simulink model "tasks"  (R2018a)
settings: Solver=FixedStepAuto  StartTime=0.0  StopTime=30  FixedStep=0.01  RelTol=1e-3
undefined symbols (not defined in the file): sigbuilder_block
settings Model: EnablePacing=on  Creator=U500304  LastModifiedBy=U500304

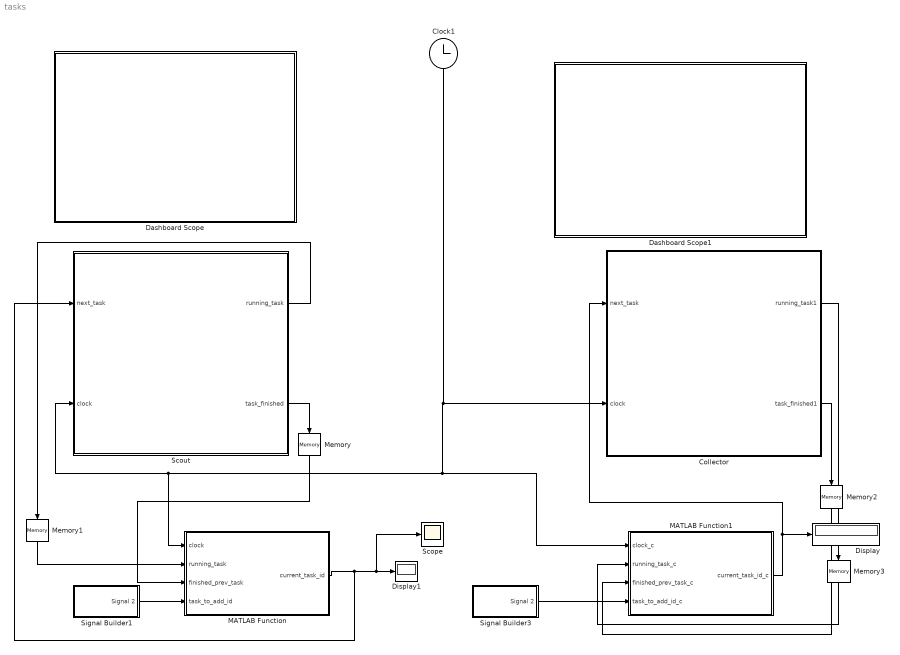
== system tasks ==
  Clock1 : Clock
  "Collector " : Subsystem
  Dashboard Scope : Subsystem  DialogController=hmiCreateDDGDialog  IsWebBlock=on  mask(MWDashboardBlock){webBlockId=7c17fb03-af4f-4b82-8f00-e62aca4ec8e7, webBlockType=sdiscope, ShowInitialText=on, HMISrcModelName=tasks}
      mask prompts: webBlockId "WebBlock Id"; webBlockType "WebBlock Type"; HMISrcModelName "Source Model"
      mask help: SimulinkHMI:dialogs:HMIScopeDialogDesc
      mask Help: helpview([docroot '/mapfiles/simulink.map'], 'hmi_scope')
      mask Display:
      | if strcmp(get_param(bdroot(gcb),'BlockDiagramType'), 'library')
      |     image([(matlabroot) '/toolbox/simulink/hmi/icons/DashboardScope.png']);
      | end
  Dashboard Scope1 : Subsystem  DialogController=hmiCreateDDGDialog  IsWebBlock=on  mask(MWDashboardBlock){webBlockId=8c902c03-5903-4973-a490-f8539d8ddacf, webBlockType=sdiscope, ShowInitialText=on, HMISrcModelName=tasks}
      mask prompts: webBlockId "WebBlock Id"; webBlockType "WebBlock Type"; HMISrcModelName "Source Model"
      mask help: SimulinkHMI:dialogs:HMIScopeDialogDesc
      mask Help: helpview([docroot '/mapfiles/simulink.map'], 'hmi_scope')
      mask Display:
      | if strcmp(get_param(bdroot(gcb),'BlockDiagramType'), 'library')
      |     image([(matlabroot) '/toolbox/simulink/hmi/icons/DashboardScope.png']);
      | end
  Display : Display
  Display1 : Display
  MATLAB Function : MATLAB Function  TreatAsAtomicUnit=on
  MATLAB Function1 : MATLAB Function  TreatAsAtomicUnit=on
  Memory{,1..3} (4 alike) : Memory
  Scope : Scope
  Scout : Subsystem
  Signal Builder1 : Subsystem  Tag=STV Subsys  LoadFcn=sigbuilder_block('load');  StartFcn=sigbuilder_block('start');  StopFcn=sigbuilder_block('stop');  ClipboardFcn=sigbuilder_block('clipboard');  mask(Sigbuilder block){tuvar=[0:10]}
      mask help: Simulink:masks:SigbuilderBlock_MD
      mask init:
      | if ~strcmp(get_param(bdroot(gcbh),'SimulationStatus'),'stopped') tuvar = sigbuilder_block('maskInit'); end
      settings: CopyFcn=sigbuilder_block('copy');  DeleteFcn=sigbuilder_block('delete');  ModelCloseFcn=sigbuilder_block('modelClose');  PreSaveFcn=sigbuilder_block('preSave');  PauseFcn=sigbuilder_block('pause');  ContinueFcn=sigbuilder_block('continue');  NameChangeFcn=sigbuilder_block('namechange');  OpenFcn=sigbuilder_block('open',[327 53.4 550.8 361.2 ]);  CloseFcn=sigbuilder_block('close');
      mask Display: plot(0, 0, 100, 100,[2, 2, 32, 32, 2], [68, 8, 8, 68, 68],[32, 2], [38, 38], [32, 19, 2],[53, 60, 44], [32, 17, 17, 2],[16, 16, 31, 31]);txt = getActiveGroup(gcbh);text(2, 100, txt,'verticalAlignment', 'top');
  Signal Builder3 : Subsystem  Tag=STV Subsys  LoadFcn=sigbuilder_block('load');  StartFcn=sigbuilder_block('start');  StopFcn=sigbuilder_block('stop');  ClipboardFcn=sigbuilder_block('clipboard');  mask(Sigbuilder block){tuvar=[0:10]}
      mask help: Simulink:masks:SigbuilderBlock_MD
      mask init:
      | if ~strcmp(get_param(bdroot(gcbh),'SimulationStatus'),'stopped') tuvar = sigbuilder_block('maskInit'); end
      settings: CopyFcn=sigbuilder_block('copy');  DeleteFcn=sigbuilder_block('delete');  ModelCloseFcn=sigbuilder_block('modelClose');  PreSaveFcn=sigbuilder_block('preSave');  PauseFcn=sigbuilder_block('pause');  ContinueFcn=sigbuilder_block('continue');  NameChangeFcn=sigbuilder_block('namechange');  OpenFcn=sigbuilder_block('open',[76.8 111.6 550.8 361.2 ]);  CloseFcn=sigbuilder_block('close');
      mask Display: plot(0, 0, 100, 100,[2, 2, 32, 32, 2], [68, 8, 8, 68, 68],[32, 2], [38, 38], [32, 19, 2],[53, 60, 44], [32, 17, 17, 2],[16, 16, 31, 31]);txt = getActiveGroup(gcbh);text(2, 100, txt,'verticalAlignment', 'top');
  wires:
  Signal Builder1/1(Signal 2) -> MATLAB Function/4(task_to_add_id)
  "Collector "/1(running_task1) -> Memory3/1
  "Collector "/2(task_finished1) -> Memory2/1
  Scout/1(running_task) -> Memory1/1
  Clock1/1 -> MATLAB Function1/1(clock_c), MATLAB Function/1(clock), Scout/2("clock "), "Collector "/2("clock ")
  MATLAB Function1/1(current_task_id_c) -> Display/1, "Collector "/1(next_task)
  Scout/2(task_finished) -> Memory/1
  Memory/1 -> MATLAB Function/3(finished_prev_task)
  MATLAB Function/1(current_task_id) -> Scout/1(next_task), Scope/1, Display1/1
  Memory1/1 -> MATLAB Function/2(running_task)
  Signal Builder3/1(Signal 2) -> MATLAB Function1/4(task_to_add_id_c)
  Memory2/1 -> MATLAB Function1/3(finished_prev_task_c)
  Memory3/1 -> MATLAB Function1/2(running_task_c)

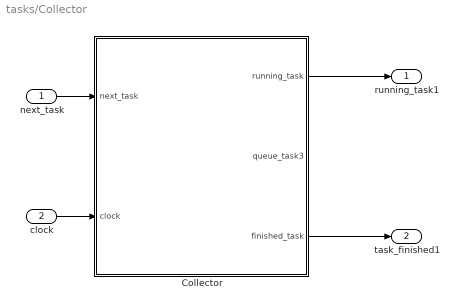
== system tasks/Collector  ==
  next_task : Inport
  "clock " : Inport  Port=2
  Collector : Stateflow chart  TreatAsAtomicUnit=on
  running_task1 : Outport
  task_finished1 : Outport  Port=2
  wires:
  next_task/1 -> Collector/1(next_task)
  "clock "/1 -> Collector/2(clock)
  Collector/3(finished_task) -> task_finished1/1
  Collector/1(running_task) -> running_task1/1

== system tasks/Dashboard Scope ==

== system tasks/Dashboard Scope1 ==

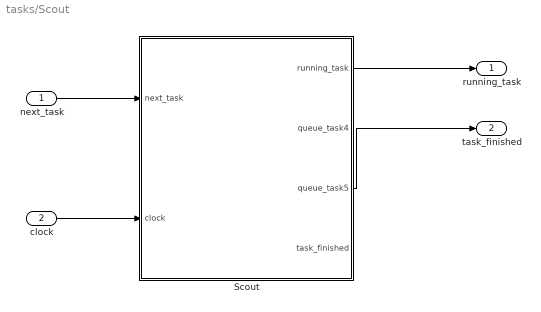
== system tasks/Scout ==
  next_task : Inport
  "clock " : Inport  Port=2
  Scout : Stateflow chart  TreatAsAtomicUnit=on
  running_task : Outport
  task_finished : Outport  Port=2
  wires:
  next_task/1 -> Scout/1(next_task)
  Scout/1(running_task) -> running_task/1
  "clock "/1 -> Scout/2(clock)
  Scout/3(" queue_task5") -> task_finished/1

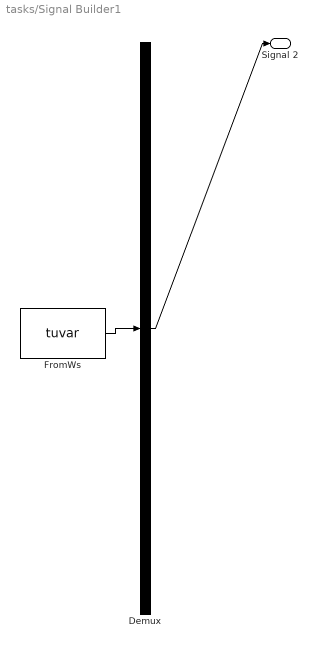
== system tasks/Signal Builder1 ==
  Demux : Demux  Tag=STV Demux  Outputs=1
  FromWs : FromWorkspace  Tag=STV FromWs  VariableName=tuvar  SampleTime=0
      SigBuilderData=|
      | common.afterFinalStr = 'Extrapolate'
      | common.sampleTime = 0
      | dataSet.timeRange = [0 10]
      | dataSet.name = 'Group 1'
      | sbobj.Groups.Name = 'Group 1'
      | sbobj.Groups.Signals.Name = 'Signal 2'
      | sbobj.Groups.Signals.XData = [0 0.5 0.5 2 2 2.5 3 3 4.5 4.5 5 5.5 6 6 8 8 8.5 9 9.5 10]
      | sbobj.Groups.Signals.YData = [0.01 0.01 1 1 0 0 0 3 3 0 0 0 0 2 2 0 0 0 0 0]
  Signal 2 : Outport  Tag=STV Outport
  wires:
  Demux/1 -> Signal 2/1
  FromWs/1 -> Demux/1

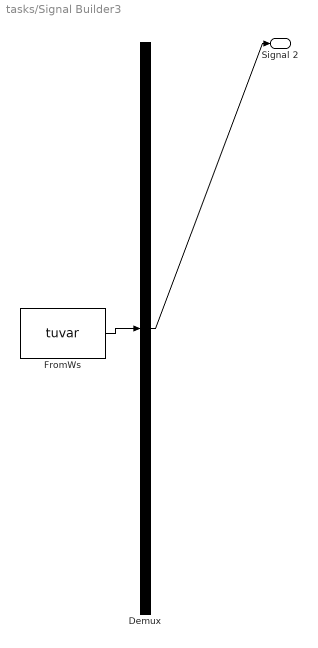
== system tasks/Signal Builder3 ==
  Demux : Demux  Tag=STV Demux  Outputs=1
  FromWs : FromWorkspace  Tag=STV FromWs  VariableName=tuvar  SampleTime=0
      SigBuilderData=|
      | common.afterFinalStr = 'Extrapolate'
      | common.sampleTime = 0
      | dataSet.timeRange = [0 10]
      | dataSet.name = 'Group 1'
      | sbobj.Groups.Name = 'Group 1'
      | sbobj.Groups.Signals.Name = 'Signal 2'
      | sbobj.Groups.Signals.XData = [0 0.5 0.5 2 2.5 3 3 4.5 4.5 5 5.5 6 6 8 8 8.5 9 9 9.5 9.5 10]
      | sbobj.Groups.Signals.YData = [0.01 0.01 0 0 0 0 4 4 0 0 0 0 0 0 0 0 0 2 2 0 0]
  Signal 2 : Outport  Tag=STV Outport
  wires:
  FromWs/1 -> Demux/1
  Demux/1 -> Signal 2/1

== matlab function tasks/MATLAB Function ==
  data: clock input; running_task input; finished_prev_task input; current_task_id output; task_to_add_id input
function current_task_id = schedule_tasklist(clock, running_task, finished_prev_task, task_to_add_id)
current_task_id = 0;

coder.updateBuildInfo('addSourceFiles','schedule_task.c');
coder.cinclude('schedule_task.h');

if (clock == 0)
    coder.ceval('initialize_tasklist');
end

coder.ceval('accept_task', task_to_add_id);
current_task = 0;
current_task = coder.ceval('next_task');

if (finished_prev_task == 1) 
    coder.ceval('remove_task', current_task);
    current_task = coder.ceval('next_task');
end
    
current_task_id = current_task;
if (running_task ~= 0 && running_task == current_task_id)
    coder.ceval('remove_task', current_task);
end  
end

== stateflow chart tasks/Scout/Scout ==
  settings: updateMethod=CONTINUOUS
  note: Placeholder for real task data
  state Schedule
    ex:
    task_finished = 0;
  state Orientation_and_Drive
    en:
    running_task = 0;
    timer = clock;
  state Generate_New_Goal
    en:
    running_task = 1;
    timer = clock;
    cost = 12;
  state Communicate_Own_Position
    en:
    running_task = 2;
    timer = clock;
    cost = 5;
  state Receive_Photo_Sensor_Readings
    en:
    running_task = 3;
    timer = clock;
    cost = 10;
  state Handle_High_Readings
    en:
    running_task = 4;
    timer = clock;
    cost = 4;
  state Communicate_Harvest_Coordinates
    en:
    running_task = 5;
    timer = clock;
    cost = 5;
  state Receive_Referee_Communication
    en:
    running_task = 6;
    timer = clock;
    cost = 7;
  (default) -> Schedule : {next_task; clock;}
  Schedule -> Orientation_and_Drive [order 3] : [next_task == 0]
  Orientation_and_Drive -> Schedule : [next_task ~= 0]{task_finished = 1;}
  Schedule -> Generate_New_Goal [order 2] : [next_task == 1]
  Generate_New_Goal -> Schedule : [clock - timer > cost]{task_finished = 1;}
  Schedule -> Communicate_Own_Position [order 1] : [next_task == 2]
  Communicate_Own_Position -> Schedule : [clock - timer > cost]{task_finished = 1;}
  Schedule -> Receive_Photo_Sensor_Readings [order 4] : [next_task == 3]
  Receive_Photo_Sensor_Readings -> Schedule : [clock - timer > cost]{task_finished = 1;}
  Schedule -> Handle_High_Readings [order 5] : [next_task == 4]
  Handle_High_Readings -> Schedule : [clock - timer > cost]{task_finished = 1;}
  Schedule -> Communicate_Harvest_Coordinates [order 6] : [next_task == 5]
  Communicate_Harvest_Coordinates -> Schedule : [clock - timer > cost]{task_finished = 1;}
  Schedule -> Receive_Referee_Communication [order 7] : [next_task == 6]
  Receive_Referee_Communication -> Schedule : [clock - timer > cost]{task_finished = 1;}
  data: next_task input; cost local; timer local; running_task output; clock input; queue_task4 output boolean; queue_task5 output boolean; task_finished output
  data timer settings: updateMethod=SF_CONTINUOUS_TIME_DATA

== matlab function tasks/MATLAB Function1 ==
  data: clock_c input; running_task_c input; finished_prev_task_c input; current_task_id_c output; task_to_add_id_c input
function current_task_id_c = schedule_tasklist(clock_c, running_task_c, finished_prev_task_c, task_to_add_id_c)
current_task_id_c = 0;

coder.updateBuildInfo('addSourceFiles','schedule_task_c.c');
coder.cinclude('schedule_task_c.h');

if (clock_c == 0)
    coder.ceval('initialize_tasklist_c');
end

coder.ceval('accept_task_c', task_to_add_id_c);
current_task_c = 0;
current_task_c = coder.ceval('next_task_c');

if (finished_prev_task_c == 1) 
    coder.ceval('remove_task_c', current_task_c);
    current_task_c = coder.ceval('next_task_c');
end
    
current_task_id_c = current_task_c;
if (running_task_c ~= 0 && running_task_c == current_task_id_c)
    coder.ceval('remove_task_c', current_task_c);
end  
end

== stateflow chart tasks/Collector /Collector ==
  settings: updateMethod=CONTINUOUS
  note: Placeholder for real task data
  state Schedule
    ex:
    finished_task = 0;
  state Orientation_and_Drive
    en:
    running_task = 0;
    timer = clock;
  state Generate_New_Goal
    en:
    running_task = 1;
    timer = clock;
    cost = 12;
  state Receive_Proximity_Sensor_Readings
    en:
    running_task = 2;
    timer = clock;
    cost = 8;
  state Handle_High_Readings
    en:
    running_task = 3;
    timer = clock;
    cost = 10;
  state Receive_Harvest_Coordinates
    en:
    running_task = 4;
    timer = clock;
    cost = 5;
  state Receive_Referee_Communication
    en:
    running_task = 5;
    timer = clock;
    cost = 5;
  (default) -> Schedule : {next_task; clock;}
  Schedule -> Orientation_and_Drive [order 2] : [next_task == 0]
  Orientation_and_Drive -> Schedule : [next_task ~= 0]
  Schedule -> Generate_New_Goal [order 1] : [next_task == 1]
  Generate_New_Goal -> Schedule : [clock - timer > cost]{finished_task = 1;}
  Schedule -> Receive_Proximity_Sensor_Readings [order 3] : [next_task == 2]
  Receive_Proximity_Sensor_Readings -> Schedule : [clock - timer > cost]{finished_task = 1;}
  Schedule -> Handle_High_Readings [order 4] : [next_task == 3]
  Handle_High_Readings -> Schedule : [clock - timer > cost]{finished_task = 1;}
  Schedule -> Receive_Harvest_Coordinates [order 5] : [next_task == 4]
  Receive_Harvest_Coordinates -> Schedule : [clock - timer > cost]{finished_task = 1;}
  Schedule -> Receive_Referee_Communication [order 6] : [next_task == 5]
  Receive_Referee_Communication -> Schedule : [clock - timer > cost]{finished_task = 1;}
  data: next_task input; cost local; timer local; running_task output; clock input; queue_task3 output boolean; finished_task output
  data timer settings: updateMethod=SF_CONTINUOUS_TIME_DATA
